simulink model "M10B39_es_V2"  (R2025a)
settings: Solver=ode23tb  StartTime=0.0  StopTime=30  FixedStep=0.001  MaxStep=0.01  RelTol=1e-3  EnableMultiTasking=on
InitFcn:
  | initAll_V2
values from neighbouring files (symbols this model uses):
  acom = 100    [initAll_V1.m]    (also in initAll_V2.m; initAll_V3.m; parameterinit.mat)
  AVm0 = [4.26082678503 4.656135219]    [parameterinit.mat]
  bcom = 50    [initAll_V1.m]    (also in initAll_V2.m; initAll_V3.m; parameterinit.mat)
  busdata = [ ... (first row only)    [PowerFlowData.m]    (also in parameterinit.mat = [1 2 3 4 5 6 7 8 9 10 11 12 ... (585 elements, 39x15)])
  commun = 0*commun    [initAll_V1.m]    (also in initAll_V2.m; initAll_V3.m; parameterinit.mat = [0  0  0; 0  0  0; 0  0  0; 0  0  0])
  Currentin_idx = [8 21 30:39]    [initAll_V2.m]    (also in parameterinit.mat = [8 21 30 31 32 33 34 35 36 37 38 39])
  DataDelay = 0.0*DataDelay    [initAll_V1.m]    (also in initAll_V2.m; initAll_V3.m; parameterinit.mat = [0  0  0; 0  0  0; 0  0  0; 0  0  0])
  ESinit =     [parameterinit.mat]
  fB = 50    [initAll.m]    (also in initAll_V1.m; initAll_V2.m; initAll_V3.m; parameterinit.mat)
  Geninit = Generator_init(opdata,SynMach_in_gidx)    [initAll.m]    (also in initAll_V1.m; initAll_V2.m; initAll_V3.m = Generator_init(opdata_all,SynMach_in_gidx1); parameterinit.mat = )
  lam = 100    [initAll_V1.m]    (also in initAll_V2.m; initAll_V3.m; parameterinit.mat)
  linedata = [1   2 0.00350  0.04110 0.69870 0.0000 ... (first row only)    [PowerFlowData.m]    (also in parameterinit.mat = [1 1 2 2 2 3 3 4 4 5 6 6 ... (276 elements, 46x6)])
  SgridB = 100    [initAll.m]    (also in initAll_V1.m; initAll_V2.m; initAll_V3.m; parameterinit.mat)
  wB = 2*pi*fB    (= 314.159265359)    [initAll.m]    (also in initAll_V1.m; initAll_V2.m; initAll_V3.m; parameterinit.mat)
  Windinit =     [parameterinit.mat]
  YY_load = [3.65450097002 -2.05705688056 0 0 0 0 0 0 0 0 0 0 ... (1521 elements, 39x39)]    [parameterinit.mat]    (also in powerflowcaculate.m = full(YY))
undefined symbols (not defined in the file or in its folder): c1, c2, c3, c4, c5, c6, cp_nom, lambda_nom, P_wind_base, Pelec_base, Pnom
libraries: spsBistableLib x12, simulink_extras x2, simulink x1
(part 2 of 7)

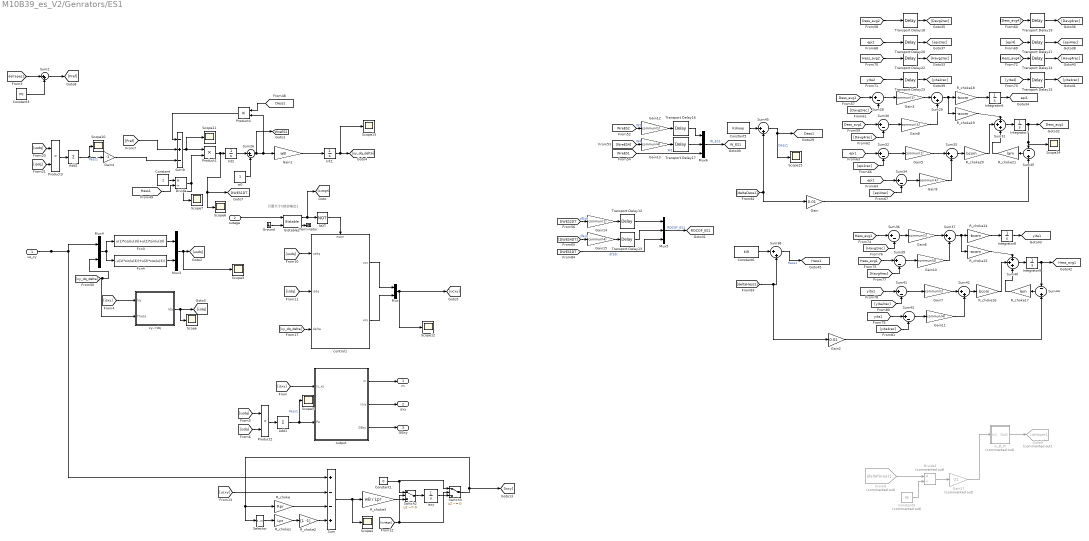
== system M10B39_es_V2/Genrators/ES1 ==
  note: 只要大于0就会输出1
  us_xy : Inport
  outage : Inport  Port=2
  " control1" : Subsystem
  Add1 : Sum  Inputs=+
  Add2 : Sum  Inputs=+
  Bistable2 : spsBistableLib/Bistable  Qpriority=Set  ic=0  Ts=0
  Constant : Constant
  Constant1 : Constant  Value=0
  Constant3 : Constant  Value=P0
  Constant4 : Constant  Commented=on  Value=fB
  Constant5 : Constant  Value=Kdroop
  Constant6 : Constant  Value=KIR
  Divide : Product  Inputs=*/
  Divide2 : Product  Commented=on  Inputs=*/
  Fcn3 : Fcn  Expr=u(1)*cos(u(3))+u(2)*sin(u(3))
  Fcn4 : Fcn  Expr=-u(1)*sin(u(3))+u(2)*cos(u(3))
  From9 : From  Commented=on  GotoTag=deltafarea1  TagVisibility=global
  Gain : Gain  Gain=0.01
  Gain1 : Gain  Gain=wB  SaturateOnIntegerOverflow=on  OutDataTypeStr=Inherit: Same as input  ParamDataTypeStr=Inherit: Same as input
  Gain{8..11,13,15} (6 alike) : Gain  Gain=commun(4)
  Gain{3,5..7,12,14} (6 alike) : Gain  Gain=commun(1)
  Gain17 : Gain  Commented=on  Gain=-21
  Gain2 : Gain  Gain=0.01
  Gain4 : Gain  Gain=-1
  Goto9 : Goto  Commented=on  GotoTag=deltapes1
  Ground : Ground
  Int1 : Integrator  InitialCondition=Dels_hvdc
  Int2 : Integrator  InitialCondition=1
  Integrator{6..9} (4 alike) : Integrator
  Isxy : Integrator  InitialCondition=[Is_xA_0 Is_yA_0]
  Mux : Mux  Inputs=2
  Mux3 : Mux  Inputs=2
  Mux4 : Mux  Inputs=2
  Mux5 : Mux  Inputs=3
  Mux6 : Mux  Inputs=3
  NOT : Logic  Operator=NOT  AllPortsSameDT=off  OutDataTypeStr=boolean
  Product1 : Product
  Product2 : Product  RndMeth=Zero
  Product3 : Product  RndMeth=Zero
  Product4 : Product
  R_choke : Gain  Gain=Rpr  SaturateOnIntegerOverflow=on  OutDataTypeStr=Inherit: Same as input  ParamDataTypeStr=Inherit: Same as input
  R_choke1 : Gain  Gain=Lpr  SaturateOnIntegerOverflow=on  OutDataTypeStr=Inherit: Same as input  ParamDataTypeStr=Inherit: Same as input
  R_choke14 : Gain  Gain=-bcom  SaturateOnIntegerOverflow=on  OutDataTypeStr=Inherit: Same as input  ParamDataTypeStr=Inherit: Same as input
  R_choke15 : Gain  Gain=-acom  SaturateOnIntegerOverflow=on  OutDataTypeStr=Inherit: Same as input  ParamDataTypeStr=Inherit: Same as input
  R_choke16 : Gain  Gain=bcom  SaturateOnIntegerOverflow=on  OutDataTypeStr=Inherit: Same as input  ParamDataTypeStr=Inherit: Same as input
  R_choke17 : Gain  Gain=lam  SaturateOnIntegerOverflow=on  OutDataTypeStr=Inherit: Same as input  ParamDataTypeStr=Inherit: Same as input
  R_choke18 : Gain  Gain=-bcom  SaturateOnIntegerOverflow=on  OutDataTypeStr=Inherit: Same as input  ParamDataTypeStr=Inherit: Same as input
  R_choke19 : Gain  Gain=-acom  SaturateOnIntegerOverflow=on  OutDataTypeStr=Inherit: Same as input  ParamDataTypeStr=Inherit: Same as input
  R_choke2 : Gain  Gain=[1 -1]  SaturateOnIntegerOverflow=on  OutDataTypeStr=Inherit: Same as input  ParamDataTypeStr=Inherit: Same as input
  R_choke20 : Gain  Gain=bcom  SaturateOnIntegerOverflow=on  OutDataTypeStr=Inherit: Same as input  ParamDataTypeStr=Inherit: Same as input
  R_choke21 : Gain  Gain=lam  SaturateOnIntegerOverflow=on  OutDataTypeStr=Inherit: Same as input  ParamDataTypeStr=Inherit: Same as input
  R_choke3 : Gain  Gain=wB / Lpr  SaturateOnIntegerOverflow=on  OutDataTypeStr=Inherit: Same as input  ParamDataTypeStr=Inherit: Same as input
  Scope{,3..7,10..15} (12 alike) : Scope
      Scope settings: ActiveDisplayYMinimum=-0.0194  ActiveDisplayYMaximum=0.04689
      Scope10 settings: ActiveDisplayYMinimum=-0.6053  ActiveDisplayYMaximum=0.06726
      Scope11 settings: ActiveDisplayYMinimum=-0.1125  ActiveDisplayYMaximum=0.0125  DataLoggingVariableName=ScopeData2
      Scope12 settings: ActiveDisplayYMinimum=0.46883  ActiveDisplayYMaximum=1.25548  DataLoggingVariableName=ScopeData3
      Scope13 settings: ActiveDisplayYMinimum=-4.33823  ActiveDisplayYMaximum=0.36599  DataLoggingVariableName=ScopeData4
      Scope14 settings: ActiveDisplayYMinimum=-0.0418  ActiveDisplayYMaximum=0.37621  DataLoggingVariableName=ScopeData2
      Scope15 settings: ActiveDisplayYMinimum=-1  ActiveDisplayYMaximum=1  DataLoggingVariableName=ScopeData3
      Scope3 settings: ActiveDisplayYMinimum=-0.14332  ActiveDisplayYMaximum=1.14443
      Scope4 settings: ActiveDisplayYMinimum=-2.8E-5  ActiveDisplayYMaximum=2.4E-5  DataLoggingVariableName=ScopeData5
      Scope5 settings: ActiveDisplayYMinimum=-0.57271  ActiveDisplayYMaximum=0.19884  DataLoggingVariableName=ScopeData7
      Scope6 settings: ActiveDisplayYMinimum=-0.00021  ActiveDisplayYMaximum=0.0004  DataLoggingVariableName=ScopeData4
      Scope7 settings: ActiveDisplayYMinimum=0.9  ActiveDisplayYMaximum=1.1  DataLoggingVariableName=ScopeData14
  Selector : Selector  InputPortWidth=2  IndexOptions=Index vector (dialog)  Indices=[2 1]  OutputSizes=1
  Sum : Sum  Inputs=+--+  SaturateOnIntegerOverflow=on
  Sum2 : Sum  Inputs=|++
  Sum{26,28,30,32,34,36,39,41,43} (9 alike) : Sum  Inputs=|+-  SaturateOnIntegerOverflow=on
  Sum{29,33,37..38,42,45} (6 alike) : Sum  Inputs=|++  SaturateOnIntegerOverflow=on
  Sum31 : Sum  Inputs=+++  SaturateOnIntegerOverflow=on
  Sum35 : Sum  Inputs=-+  SaturateOnIntegerOverflow=on
  Sum40 : Sum  Inputs=+++  SaturateOnIntegerOverflow=on
  Sum44 : Sum  Inputs=-+  SaturateOnIntegerOverflow=on
  Sum9 : Sum  Inputs=-+-  SaturateOnIntegerOverflow=on
  Switch2 : Switch  Criteria=u2 ~= 0  Threshold=0.5  InputSameDT=off
  Switch3 : Switch  Criteria=u2 ~= 0  Threshold=0.5  InputSameDT=off
  Terminator : Terminator
  Transport Delay{12,16,18,20,22..23} (6 alike) : TransportDelay  DelayTime=DataDelay(2,1)
  Transport Delay{13..15,17,19,21} (6 alike) : TransportDelay  DelayTime=DataDelay(4,2)
  in_D_PI : Subsystem  Commented=on  mask{KP_=0.1, KI_=0.1, Upper_limit=inf, Lower_limit=-inf, Upper_saturation_limit=inf, Lower_saturation_limit=-inf, integrator_init=Md_A_0}
      mask prompts: KP_ "比例系数P"; KI_ "积分系数I"; Upper_limit "限幅上限"; Lower_limit "限幅下限"; Upper_saturation_limit "积分饱和上限"; Lower_saturation_limit "积分饱和下限"; integrator_init "积分初始值"
      mask DialogControl Container4 Prompt: 控制参数
      mask DialogControl Container5 Prompt: 初始值
      mask Display: disp('PI')
  output : Subsystem
  w0 : Constant
  xy->dq : Subsystem
  m : Outport
  isxy : Outport  Port=2
  GBxy : Outport  Port=3
  tag scope: DWES1DT=global, Dess1=global, Dess_avg1=global, Hess1=global, Hess_avg1=global, ROCOF_ES1=global, W_ES1=global, WreES1=global, epi1=global, yita1=global
  wires:
  Selector/1 -> R_choke1/1
  Sum/1 -> Scope4/1, R_choke3/1
  R_choke3/1 -> Switch2/3
  Ground/1 -> Bistable2/2
  R_choke2/1 -> Sum/4
  R_choke/1 -> Sum/3
  [ucxy] -> Sum/2
  output/1(m) -> m/1
  NOT/1 -> " control1"/Enable
  R_choke1/1 -> R_choke2/1
  Bistable2/1 -> NOT/1, [outage]
  Isxy/1 -> Switch3/3
  [isxy] -> xy->dq/1(Ixy)
  [isxy] -> output/1(is_xy)
  output/2(isxy) -> isxy/1
  [xy_dq_delta] -> " control1"/3(delta)
  xy->dq/1(Idq) -> [isdq], Scope/1
  Bistable2/2 -> Terminator/1
  outage/1 -> Bistable2/1
  [outage] -> Switch2/2, Switch3/2
  [isdq] -> " control1"/2(isdq)
  " control1"/1(ucx) -> Mux/1
  Switch2/1 -> Isxy/1
  Switch3/1 -> R_choke/1, Selector/1, [isxy]
  Mux/1 -> Scope12/1, [ucxy]
  [usdq] -> " control1"/1(usdq)
  output/3(GBxy) -> GBxy/1
  Constant1/1 -> Switch2/1, Switch3/1
  " control1"/2(ucy) -> Mux/2
  [usdq] -> Product2/1
  Add1/1 -> Scope5/1, output/2(Pe)  "Pess1"
  Product2/1 -> Add1/1
  [isdq] -> Product2/2
  Product1/1 -> Scope6/1, [DWES1DT], Int2/1
  Sum26/1 -> [WreES1], Product4/2, Gain1/1
  Int2/1 -> Sum26/1
  w0/1 -> Sum26/2
  Sum9/1 -> Product1/1, Scope11/1
  Constant/1 -> Divide/1
  Divide/1 -> Product1/2, Scope7/1
  [Hess1] -> Divide/2
  us_xy/1 -> Mux4/1, Sum/1
  Fcn3/1 -> Mux3/1
  Fcn4/1 -> Mux3/2
  Mux4/1 -> Fcn3/1, Fcn4/1
  [xy_dq_delta] -> Mux4/2, xy->dq/2(Theta)
  Mux3/1 -> Scope3/1, [usdq]
  Gain4/1 -> Sum9/3
  Product4/1 -> Sum9/1
  Int1/1 -> Scope13/1, [xy_dq_delta]
  Add2/1 -> Gain4/1, Scope10/1  "Pess1"
  [usdq] -> Product3/1
  [isdq] -> Product3/2
  Product3/1 -> Add2/1
  Transport Delay19/1 -> [Davg4rec]
  R_choke20/1 -> Sum31/2
  R_choke19/1 -> Sum31/1
  [Dess_avg1] -> Sum28/1
  Transport Delay13/1 -> Mux5/2
  Transport Delay12/1 -> Mux5/1
  [Dess_avg1] -> Sum30/1
  Mux6/1 -> [W_ES1]  "W_ES1"
  [WreES1] -> Mux6/3  "W1"
  Sum38/1 -> [Hess1]  "Hess1"
  Constant5/1 -> Sum45/1
  Sum45/1 -> Scope15/1, [Dess1]  "Dess1"
  Constant6/1 -> Sum38/1
  [epi1] -> Sum34/1
  R_choke21/1 -> Sum31/3
  Integrator6/1 -> [epi1]
  Sum35/1 -> R_choke21/1
  Sum31/1 -> Integrator7/1
  Integrator7/1 -> [Dess_avg1], Scope14/1, Sum35/1
  Transport Delay21/1 -> [epi4rec]
  [epi2] -> Transport Delay20/1
  [epi4rec] -> Sum34/2
  [DWES1DT] -> Mux5/3  "df1dt"
  [Davg4rec] -> Sum30/2
  [yita2rec] -> Sum41/2
  [yita1] -> Sum41/1
  Sum40/1 -> Integrator9/1
  [deltaDess1] -> Sum45/2, Gain/1
  R_choke18/1 -> Integrator6/1
  [Havg4rec] -> Sum39/2
  [epi1] -> Sum32/1
  [Havg2rec] -> Sum36/2
  Sum42/1 -> R_choke16/1
  [Dess_avg2] -> Transport Delay18/1
  Transport Delay20/1 -> [epi2rec]
  Transport Delay14/1 -> [Havg4rec]
  [Hess_avg1] -> Sum39/1
  Mux5/1 -> [ROCOF_ES1]  "ROCOF_ES1"
  Integrator9/1 -> [Hess_avg1], Sum44/1
  Sum29/1 -> R_choke19/1, R_choke18/1
  [Davg2rec] -> Sum28/2
  [yita2] -> Transport Delay23/1
  Sum37/1 -> R_choke15/1, R_choke14/1
  R_choke14/1 -> Integrator8/1
  Integrator8/1 -> [yita1]
  Transport Delay18/1 -> [Davg2rec]
  R_choke17/1 -> Sum40/3
  Transport Delay17/1 -> Mux6/2
  R_choke15/1 -> Sum40/1
  R_choke16/1 -> Sum40/2
  [Hess_avg1] -> Sum36/1
  [deltaHess1] -> Sum38/2, Gain2/1
  Sum44/1 -> R_choke17/1
  Sum33/1 -> R_choke20/1
  Transport Delay23/1 -> [yita2rec]
  Transport Delay16/1 -> Mux6/1
  [epi2rec] -> Sum32/2
  Transport Delay22/1 -> [Havg2rec]
  Transport Delay15/1 -> [yita4rec]
  [Hess_avg2] -> Transport Delay22/1
  [Dess1] -> Product4/1
  Gain1/1 -> Int1/1
  [yita4rec] -> Sum43/2
  [yita1] -> Sum43/1
  Gain/1 -> Sum35/2
  Gain2/1 -> Sum44/2
  [Dess_avg4] -> Transport Delay19/1
  [epi4] -> Transport Delay21/1
  [Hess_avg4] -> Transport Delay14/1
  [yita4] -> Transport Delay15/1
  [WreES2] -> Gain12/1  "W2"
  Gain12/1 -> Transport Delay16/1
  [WreES4] -> Gain13/1  "W4"
  Gain13/1 -> Transport Delay17/1
  [DWES2DT] -> Gain14/1  "df2dt"
  Gain14/1 -> Transport Delay12/1
  [DWES4DT] -> Gain15/1  "df4dt"
  Gain15/1 -> Transport Delay13/1
  Gain3/1 -> Sum29/1
  Sum28/1 -> Gain3/1
  Gain5/1 -> Sum33/1
  Sum32/1 -> Gain5/1
  Sum36/1 -> Gain6/1
  Gain6/1 -> Sum37/1
  Gain7/1 -> Sum42/1
  Sum41/1 -> Gain7/1
  Sum30/1 -> Gain8/1
  Gain8/1 -> Sum29/2
  Sum34/1 -> Gain9/1
  Gain9/1 -> Sum33/2
  Sum39/1 -> Gain10/1
  Gain10/1 -> Sum37/2
  Sum43/1 -> Gain11/1
  Gain11/1 -> Sum42/2
  [deltapes1] -> Sum2/1
  Sum2/1 -> [Pref]
  Constant3/1 -> Sum2/2
  [Pref] -> Sum9/2
  Divide2/1 -> Gain17/1
  Constant4/1 -> Divide2/2
  From9/1 -> Divide2/1
  in_D_PI/1(Out1) -> Goto9/1
  Gain17/1 -> in_D_PI/1(In1)

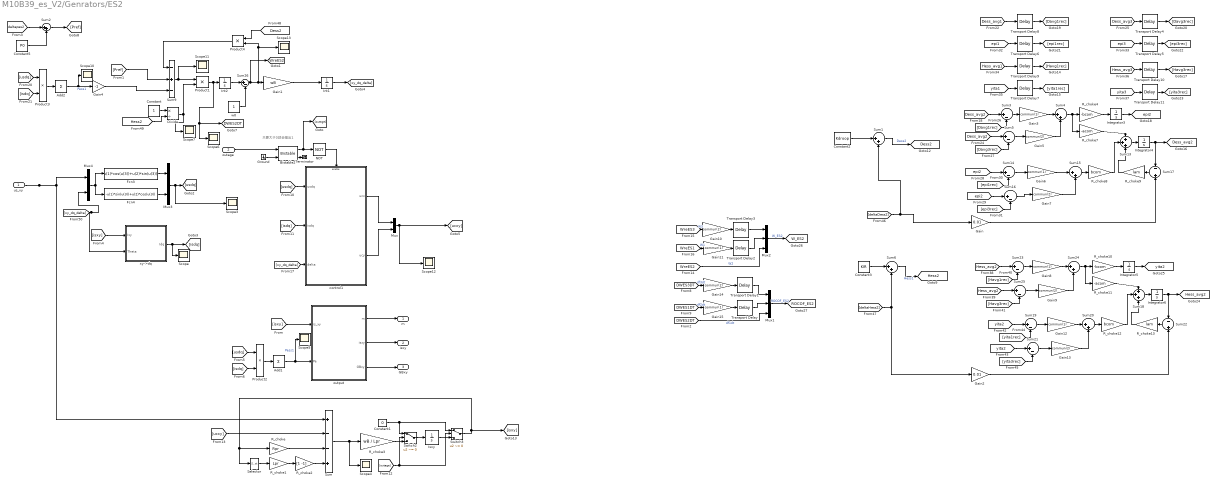
== system M10B39_es_V2/Genrators/ES2 ==
  note: 只要大于0就会输出1
  us_xy : Inport
  outage : Inport  Port=2
  " control1" : Subsystem
  Add1 : Sum  Inputs=+
  Add2 : Sum  Inputs=+
  Bistable2 : spsBistableLib/Bistable  Qpriority=Set  ic=0  Ts=0
  Constant : Constant
  Constant1 : Constant  Value=0
  Constant2 : Constant  Value=Kdroop
  Constant3 : Constant  Value=KIR
  Constant5 : Constant  Value=P0
  Divide : Product  Inputs=*/
  Fcn3 : Fcn  Expr=u(1)*cos(u(3))+u(2)*sin(u(3))
  Fcn4 : Fcn  Expr=-u(1)*sin(u(3))+u(2)*cos(u(3))
  Gain : Gain  Gain=0.01
  Gain1 : Gain  Gain=wB  SaturateOnIntegerOverflow=on  OutDataTypeStr=Inherit: Same as input  ParamDataTypeStr=Inherit: Same as input
  Gain{5,7,9..10,13..14} (6 alike) : Gain  Gain=commun(2)
  Gain{3,6,8,11..12,15} (6 alike) : Gain  Gain=commun(1)
  Gain2 : Gain  Gain=0.01
  Gain4 : Gain  Gain=-1
  Ground : Ground
  Int1 : Integrator  InitialCondition=Dels_hvdc
  Int2 : Integrator  InitialCondition=1
  Integrator{3..6} (4 alike) : Integrator
  Isxy : Integrator  InitialCondition=[Is_xA_0 Is_yA_0]
  Mux : Mux  Inputs=2
  Mux1 : Mux  Inputs=3
  Mux2 : Mux  Inputs=3
  Mux3 : Mux  Inputs=2
  Mux4 : Mux  Inputs=2
  NOT : Logic  Operator=NOT  AllPortsSameDT=off  OutDataTypeStr=boolean
  Product1 : Product
  Product2 : Product  RndMeth=Zero
  Product3 : Product  RndMeth=Zero
  Product4 : Product
  R_choke : Gain  Gain=Rpr  SaturateOnIntegerOverflow=on  OutDataTypeStr=Inherit: Same as input  ParamDataTypeStr=Inherit: Same as input
  R_choke1 : Gain  Gain=Lpr  SaturateOnIntegerOverflow=on  OutDataTypeStr=Inherit: Same as input  ParamDataTypeStr=Inherit: Same as input
  R_choke10 : Gain  Gain=-bcom  SaturateOnIntegerOverflow=on  OutDataTypeStr=Inherit: Same as input  ParamDataTypeStr=Inherit: Same as input
  R_choke11 : Gain  Gain=-acom  SaturateOnIntegerOverflow=on  OutDataTypeStr=Inherit: Same as input  ParamDataTypeStr=Inherit: Same as input
  R_choke12 : Gain  Gain=bcom  SaturateOnIntegerOverflow=on  OutDataTypeStr=Inherit: Same as input  ParamDataTypeStr=Inherit: Same as input
  R_choke13 : Gain  Gain=lam  SaturateOnIntegerOverflow=on  OutDataTypeStr=Inherit: Same as input  ParamDataTypeStr=Inherit: Same as input
  R_choke2 : Gain  Gain=[1 -1]  SaturateOnIntegerOverflow=on  OutDataTypeStr=Inherit: Same as input  ParamDataTypeStr=Inherit: Same as input
  R_choke3 : Gain  Gain=wB / Lpr  SaturateOnIntegerOverflow=on  OutDataTypeStr=Inherit: Same as input  ParamDataTypeStr=Inherit: Same as input
  R_choke4 : Gain  Gain=-bcom  SaturateOnIntegerOverflow=on  OutDataTypeStr=Inherit: Same as input  ParamDataTypeStr=Inherit: Same as input
  R_choke7 : Gain  Gain=-acom  SaturateOnIntegerOverflow=on  OutDataTypeStr=Inherit: Same as input  ParamDataTypeStr=Inherit: Same as input
  R_choke8 : Gain  Gain=bcom  SaturateOnIntegerOverflow=on  OutDataTypeStr=Inherit: Same as input  ParamDataTypeStr=Inherit: Same as input
  R_choke9 : Gain  Gain=lam  SaturateOnIntegerOverflow=on  OutDataTypeStr=Inherit: Same as input  ParamDataTypeStr=Inherit: Same as input
  Scope{,3..7,10..13} (10 alike) : Scope
      Scope settings: ActiveDisplayYMinimum=-0.0194  ActiveDisplayYMaximum=0.04689
      Scope10 settings: ActiveDisplayYMinimum=-0.00511  ActiveDisplayYMaximum=0.046
      Scope11 settings: ActiveDisplayYMinimum=-0.1125  ActiveDisplayYMaximum=0.0125  DataLoggingVariableName=ScopeData2
      Scope12 settings: ActiveDisplayYMinimum=0.46883  ActiveDisplayYMaximum=1.25548  DataLoggingVariableName=ScopeData3
      Scope13 settings: ActiveDisplayYMinimum=-0.0063  ActiveDisplayYMaximum=0.05669  DataLoggingVariableName=ScopeData4
      Scope3 settings: ActiveDisplayYMinimum=-0.12696  ActiveDisplayYMaximum=1.14248
      Scope4 settings: ActiveDisplayYMinimum=-2.8E-5  ActiveDisplayYMaximum=2.4E-5  DataLoggingVariableName=ScopeData5
      Scope5 settings: ActiveDisplayYMinimum=-0.00823  ActiveDisplayYMaximum=0.07404  DataLoggingVariableName=ScopeData7
      Scope6 settings: ActiveDisplayYMinimum=-0.00105  ActiveDisplayYMaximum=0.00091  DataLoggingVariableName=ScopeData4
      Scope7 settings: ActiveDisplayYMinimum=0.9  ActiveDisplayYMaximum=1.1  DataLoggingVariableName=ScopeData14
  Selector : Selector  InputPortWidth=2  IndexOptions=Index vector (dialog)  Indices=[2 1]  OutputSizes=1
  Sum : Sum  Inputs=+--+  SaturateOnIntegerOverflow=on
  Sum{1,4,6,15,20,24} (6 alike) : Sum  Inputs=|++  SaturateOnIntegerOverflow=on
  Sum13 : Sum  Inputs=+++  SaturateOnIntegerOverflow=on
  Sum{3,5,14,16,19,21,23,25..26} (9 alike) : Sum  Inputs=|+-  SaturateOnIntegerOverflow=on
  Sum17 : Sum  Inputs=-+  SaturateOnIntegerOverflow=on
  Sum18 : Sum  Inputs=+++  SaturateOnIntegerOverflow=on
  Sum2 : Sum  Inputs=|++
  Sum22 : Sum  Inputs=-+  SaturateOnIntegerOverflow=on
  Sum9 : Sum  Inputs=-+-  SaturateOnIntegerOverflow=on
  Switch2 : Switch  Criteria=u2 ~= 0  Threshold=0.5  InputSameDT=off
  Switch3 : Switch  Criteria=u2 ~= 0  Threshold=0.5  InputSameDT=off
  Terminator : Terminator
  Transport Delay{,2,6..9} (6 alike) : TransportDelay  DelayTime=DataDelay(1,2)
  Transport Delay{1,3..5,10..11} (6 alike) : TransportDelay  DelayTime=DataDelay(3,1)
  output : Subsystem
  w0 : Constant
  xy->dq : Subsystem
  m : Outport
  isxy : Outport  Port=2
  GBxy : Outport  Port=3
  tag scope: DWES2DT=global, Dess2=global, Dess_avg2=global, Hess2=global, Hess_avg2=global, ROCOF_ES2=global, W_ES2=global, WreES2=global, epi2=global, yita2=global
  wires:
  Selector/1 -> R_choke1/1
  Sum/1 -> Scope4/1, R_choke3/1
  R_choke3/1 -> Switch2/3
  Ground/1 -> Bistable2/2
  R_choke2/1 -> Sum/4
  R_choke/1 -> Sum/3
  [ucxy] -> Sum/2
  output/1(m) -> m/1
  NOT/1 -> " control1"/Enable
  R_choke1/1 -> R_choke2/1
  Bistable2/1 -> NOT/1, [outage]
  Isxy/1 -> Switch3/3
  [isxy] -> xy->dq/1(Ixy)
  [isxy] -> output/1(is_xy)
  output/2(isxy) -> isxy/1
  [xy_dq_delta] -> " control1"/3(delta)
  xy->dq/1(Idq) -> [isdq], Scope/1
  Bistable2/2 -> Terminator/1
  outage/1 -> Bistable2/1
  [outage] -> Switch2/2, Switch3/2
  [isdq] -> " control1"/2(isdq)
  " control1"/1(ucx) -> Mux/1
  Switch2/1 -> Isxy/1
  Switch3/1 -> R_choke/1, Selector/1, [isxy]
  Mux/1 -> Scope12/1, [ucxy]
  [usdq] -> " control1"/1(usdq)
  output/3(GBxy) -> GBxy/1
  Constant1/1 -> Switch2/1, Switch3/1
  " control1"/2(ucy) -> Mux/2
  [usdq] -> Product2/1
  Add1/1 -> Scope5/1, output/2(Pe)  "Pess1"
  Product2/1 -> Add1/1
  [isdq] -> Product2/2
  Product1/1 -> Scope6/1, [DWES2DT], Int2/1
  Sum26/1 -> [WreES2], Scope13/1, Product4/2, Gain1/1
  Int2/1 -> Sum26/1
  w0/1 -> Sum26/2
  Sum9/1 -> Product1/1, Scope11/1
  Constant/1 -> Divide/1
  Divide/1 -> Product1/2, Scope7/1
  [Hess2] -> Divide/2
  us_xy/1 -> Mux4/1, Sum/1
  Fcn3/1 -> Mux3/1
  Fcn4/1 -> Mux3/2
  Mux4/1 -> Fcn3/1, Fcn4/1
  [xy_dq_delta] -> Mux4/2, xy->dq/2(Theta)
  Mux3/1 -> Scope3/1, [usdq]
  Gain4/1 -> Sum9/3
  Product4/1 -> Sum9/1
  Int1/1 -> [xy_dq_delta]
  Add2/1 -> Gain4/1, Scope10/1  "Pess1"
  [usdq] -> Product3/1
  [isdq] -> Product3/2
  Product3/1 -> Add2/1
  [Dess2] -> Product4/1
  Gain1/1 -> Int1/1
  [Davg3rec] -> Sum5/2
  R_choke7/1 -> Sum13/1
  [yita1rec] -> Sum19/2
  Transport Delay/1 -> Mux1/2
  R_choke8/1 -> Sum13/2
  [Dess_avg2] -> Sum5/1
  [Dess_avg2] -> Sum3/1
  Transport Delay9/1 -> [Havg1rec]
  [Davg1rec] -> Sum3/2
  Transport Delay6/1 -> [epi1rec]
  [WreES2] -> Mux2/3  "W2"
  Integrator3/1 -> [epi2]
  [epi1rec] -> Sum14/2
  Transport Delay5/1 -> [epi3rec]
  Mux1/1 -> [ROCOF_ES2]  "ROCOF_ES2"
  Sum20/1 -> R_choke12/1
  Transport Delay4/1 -> [Davg3rec]
  [yita2] -> Sum21/1
  Transport Delay7/1 -> [yita1rec]
  Transport Delay3/1 -> Mux2/1
  Sum17/1 -> R_choke9/1
  [deltaDess2] -> Gain/1, Sum1/2
  [Hess_avg2] -> Sum25/1
  Sum13/1 -> Integrator4/1
  R_choke10/1 -> Integrator5/1
  Sum15/1 -> R_choke8/1
  R_choke9/1 -> Sum13/3
  Constant3/1 -> Sum6/1
  Integrator4/1 -> [Dess_avg2], Sum17/1
  [epi2] -> Sum16/1
  [deltaHess2] -> Sum6/2, Gain2/1
  Transport Delay10/1 -> [Havg3rec]
  [epi3rec] -> Sum16/2
  Sum24/1 -> R_choke11/1, R_choke10/1
  [DWES2DT] -> Mux1/3  "df1dt"
  Sum6/1 -> [Hess2]  "Hess1"
  [yita2] -> Sum19/1
  Transport Delay1/1 -> Mux1/1
  [epi2] -> Sum14/1
  R_choke12/1 -> Sum18/2
  [Hess_avg2] -> Sum23/1
  R_choke11/1 -> Sum18/1
  Transport Delay2/1 -> Mux2/2
  R_choke4/1 -> Integrator3/1
  Mux2/1 -> [W_ES2]  "W_ES2"
  Sum4/1 -> R_choke7/1, R_choke4/1
  [yita3rec] -> Sum21/2
  [Havg1rec] -> Sum23/2
  [Havg3rec] -> Sum25/2
  Transport Delay11/1 -> [yita3rec]
  Sum22/1 -> R_choke13/1
  Integrator6/1 -> [Hess_avg2], Sum22/1
  Sum18/1 -> Integrator6/1
  Integrator5/1 -> [yita2]
  R_choke13/1 -> Sum18/3
  Transport Delay8/1 -> [Davg1rec]
  Sum1/1 -> [Dess2]  "Dess2"
  Constant2/1 -> Sum1/1
  Gain/1 -> Sum17/2
  Gain2/1 -> Sum22/2
  [Dess_avg1] -> Transport Delay8/1
  [epi1] -> Transport Delay6/1
  [Hess_avg1] -> Transport Delay9/1
  [yita1] -> Transport Delay7/1
  [Dess_avg3] -> Transport Delay4/1
  [epi3] -> Transport Delay5/1
  [Hess_avg3] -> Transport Delay10/1
  [yita3] -> Transport Delay11/1
  [WreES3] -> Gain10/1  "W3"
  Gain10/1 -> Transport Delay3/1
  [WreES1] -> Gain11/1  "W1"
  Gain11/1 -> Transport Delay2/1
  [DWES3DT] -> Gain14/1  "df3dt"
  Gain14/1 -> Transport Delay1/1
  [DWES1DT] -> Gain15/1  "df2dt"
  Gain15/1 -> Transport Delay/1
  Gain3/1 -> Sum4/1
  Sum3/1 -> Gain3/1
  Sum5/1 -> Gain5/1
  Gain5/1 -> Sum4/2
  Gain6/1 -> Sum15/1
  Sum14/1 -> Gain6/1
  Sum16/1 -> Gain7/1
  Gain7/1 -> Sum15/2
  Sum23/1 -> Gain8/1
  Gain8/1 -> Sum24/1
  Sum25/1 -> Gain9/1
  Gain9/1 -> Sum24/2
  Gain12/1 -> Sum20/1
  Sum19/1 -> Gain12/1
  Sum21/1 -> Gain13/1
  Gain13/1 -> Sum20/2
  Constant5/1 -> Sum2/2
  Sum2/1 -> [Pref]
  [deltapes2] -> Sum2/1
  [Pref] -> Sum9/2

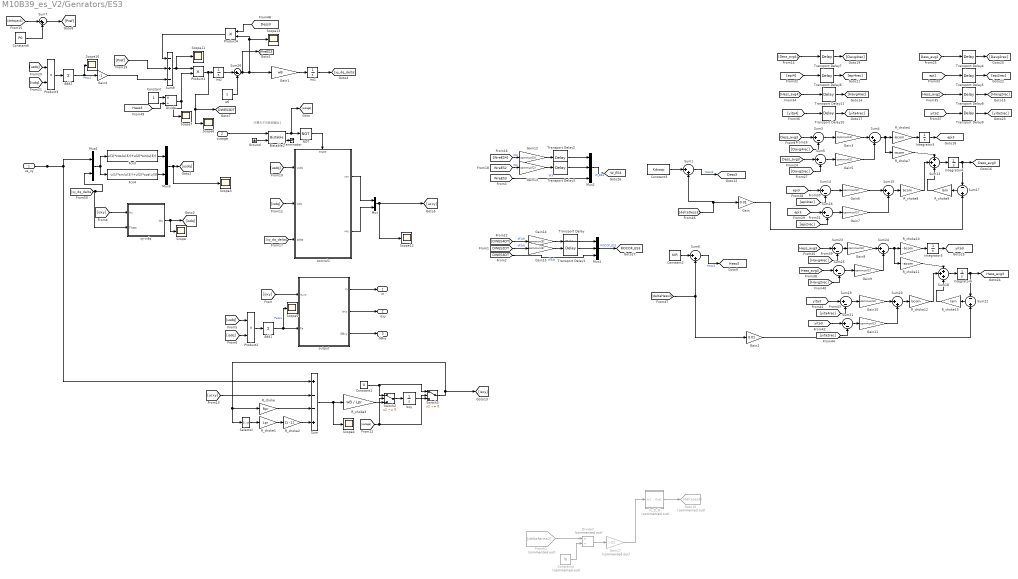
== system M10B39_es_V2/Genrators/ES3 ==
  note: 只要大于0就会输出1
  us_xy : Inport
  outage : Inport  Port=2
  " control1" : Subsystem
  Add1 : Sum  Inputs=+
  Add2 : Sum  Inputs=+
  Bistable2 : spsBistableLib/Bistable  Qpriority=Set  ic=0  Ts=0
  Constant : Constant
  Constant1 : Constant  Value=0
  Constant2 : Constant  Value=KIR
  Constant3 : Constant  Value=Kdroop
  Constant4 : Constant  Commented=on  Value=fB
  Constant6 : Constant  Value=P0
  Divide : Product  Inputs=*/
  Divide2 : Product  Commented=on  Inputs=*/
  Fcn3 : Fcn  Expr=u(1)*cos(u(3))+u(2)*sin(u(3))
  Fcn4 : Fcn  Expr=-u(1)*sin(u(3))+u(2)*cos(u(3))
  From51 : From  Commented=on  GotoTag=deltafarea2  TagVisibility=global
  Gain : Gain  Gain=0.01
  Gain1 : Gain  Gain=wB  SaturateOnIntegerOverflow=on  OutDataTypeStr=Inherit: Same as input  ParamDataTypeStr=Inherit: Same as input
  Gain{3,6,8,10,12,14} (6 alike) : Gain  Gain=commun(3)
  Gain{5,7,9,11,13,15} (6 alike) : Gain  Gain=commun(2)
  Gain17 : Gain  Commented=on  Gain=-21
  Gain2 : Gain  Gain=0.01
  Gain4 : Gain  Gain=-1
  Goto10 : Goto  Commented=on  GotoTag=deltapes3
  Ground : Ground
  Int1 : Integrator  InitialCondition=Dels_hvdc
  Int2 : Integrator  InitialCondition=1
  Integrator{3..6} (4 alike) : Integrator
  Isxy : Integrator  InitialCondition=[Is_xA_0 Is_yA_0]
  Mux : Mux  Inputs=2
  Mux1 : Mux  Inputs=3
  Mux2 : Mux  Inputs=3
  Mux3 : Mux  Inputs=2
  Mux4 : Mux  Inputs=2
  NOT : Logic  Operator=NOT  AllPortsSameDT=off  OutDataTypeStr=boolean
  Product1 : Product
  Product2 : Product  RndMeth=Zero
  Product3 : Product  RndMeth=Zero
  Product4 : Product
  R_choke : Gain  Gain=Rpr  SaturateOnIntegerOverflow=on  OutDataTypeStr=Inherit: Same as input  ParamDataTypeStr=Inherit: Same as input
  R_choke1 : Gain  Gain=Lpr  SaturateOnIntegerOverflow=on  OutDataTypeStr=Inherit: Same as input  ParamDataTypeStr=Inherit: Same as input
  R_choke10 : Gain  Gain=-bcom  SaturateOnIntegerOverflow=on  OutDataTypeStr=Inherit: Same as input  ParamDataTypeStr=Inherit: Same as input
  R_choke11 : Gain  Gain=-acom  SaturateOnIntegerOverflow=on  OutDataTypeStr=Inherit: Same as input  ParamDataTypeStr=Inherit: Same as input
  R_choke12 : Gain  Gain=bcom  SaturateOnIntegerOverflow=on  OutDataTypeStr=Inherit: Same as input  ParamDataTypeStr=Inherit: Same as input
  R_choke13 : Gain  Gain=lam  SaturateOnIntegerOverflow=on  OutDataTypeStr=Inherit: Same as input  ParamDataTypeStr=Inherit: Same as input
  R_choke2 : Gain  Gain=[1 -1]  SaturateOnIntegerOverflow=on  OutDataTypeStr=Inherit: Same as input  ParamDataTypeStr=Inherit: Same as input
  R_choke3 : Gain  Gain=wB / Lpr  SaturateOnIntegerOverflow=on  OutDataTypeStr=Inherit: Same as input  ParamDataTypeStr=Inherit: Same as input
  R_choke4 : Gain  Gain=-bcom  SaturateOnIntegerOverflow=on  OutDataTypeStr=Inherit: Same as input  ParamDataTypeStr=Inherit: Same as input
  R_choke7 : Gain  Gain=-acom  SaturateOnIntegerOverflow=on  OutDataTypeStr=Inherit: Same as input  ParamDataTypeStr=Inherit: Same as input
  R_choke8 : Gain  Gain=bcom  SaturateOnIntegerOverflow=on  OutDataTypeStr=Inherit: Same as input  ParamDataTypeStr=Inherit: Same as input
  R_choke9 : Gain  Gain=lam  SaturateOnIntegerOverflow=on  OutDataTypeStr=Inherit: Same as input  ParamDataTypeStr=Inherit: Same as input
  Scope{,3..7,10..13} (10 alike) : Scope
      Scope settings: ActiveDisplayYMinimum=-0.0194  ActiveDisplayYMaximum=0.04689
      Scope10 settings: ActiveDisplayYMinimum=-0.00511  ActiveDisplayYMaximum=0.046
      Scope11 settings: ActiveDisplayYMinimum=-0.1125  ActiveDisplayYMaximum=0.0125  DataLoggingVariableName=ScopeData2
      Scope12 settings: ActiveDisplayYMinimum=0.46883  ActiveDisplayYMaximum=1.25548  DataLoggingVariableName=ScopeData3
      Scope13 settings: ActiveDisplayYMinimum=-0.00656  ActiveDisplayYMaximum=0.05904  DataLoggingVariableName=ScopeData4
      Scope3 settings: ActiveDisplayYMinimum=-0.12696  ActiveDisplayYMaximum=1.14248
      Scope4 settings: ActiveDisplayYMinimum=-2.8E-5  ActiveDisplayYMaximum=2.4E-5  DataLoggingVariableName=ScopeData5
      Scope5 settings: ActiveDisplayYMinimum=-0.00823  ActiveDisplayYMaximum=0.07404  DataLoggingVariableName=ScopeData7
      Scope6 settings: ActiveDisplayYMinimum=-4.9E-5  ActiveDisplayYMaximum=-0  DataLoggingVariableName=ScopeData4
      Scope7 settings: ActiveDisplayYMinimum=0.9  ActiveDisplayYMaximum=1.1  DataLoggingVariableName=ScopeData14
  Selector : Selector  InputPortWidth=2  IndexOptions=Index vector (dialog)  Indices=[2 1]  OutputSizes=1
  Sum : Sum  Inputs=+--+  SaturateOnIntegerOverflow=on
  Sum{1,4,6,15,20,24} (6 alike) : Sum  Inputs=|++  SaturateOnIntegerOverflow=on
  Sum13 : Sum  Inputs=+++  SaturateOnIntegerOverflow=on
  Sum{3,5,14,16,19,21,23,25..26} (9 alike) : Sum  Inputs=|+-  SaturateOnIntegerOverflow=on
  Sum17 : Sum  Inputs=-+  SaturateOnIntegerOverflow=on
  Sum18 : Sum  Inputs=+++  SaturateOnIntegerOverflow=on
  Sum22 : Sum  Inputs=-+  SaturateOnIntegerOverflow=on
  Sum7 : Sum  Inputs=|++
  Sum9 : Sum  Inputs=-+-  SaturateOnIntegerOverflow=on
  Switch2 : Switch  Criteria=u2 ~= 0  Threshold=0.5  InputSameDT=off
  Switch3 : Switch  Criteria=u2 ~= 0  Threshold=0.5  InputSameDT=off
  Terminator : Terminator
  Transport Delay{,2,6..7,10..11} (6 alike) : TransportDelay  DelayTime=DataDelay(4,1)
  Transport Delay{1,3..5,8..9} (6 alike) : TransportDelay  DelayTime=DataDelay(2,2)
  in_D_PI : Subsystem  Commented=on  mask{KP_=0.1, KI_=0.1, Upper_limit=inf, Lower_limit=-inf, Upper_saturation_limit=inf, Lower_saturation_limit=-inf, integrator_init=Md_A_0}
      mask prompts: KP_ "比例系数P"; KI_ "积分系数I"; Upper_limit "限幅上限"; Lower_limit "限幅下限"; Upper_saturation_limit "积分饱和上限"; Lower_saturation_limit "积分饱和下限"; integrator_init "积分初始值"
      mask DialogControl Container4 Prompt: 控制参数
      mask DialogControl Container5 Prompt: 初始值
      mask Display: disp('PI')
  output : Subsystem
  w0 : Constant
  xy->dq : Subsystem
  m : Outport
  isxy : Outport  Port=2
  GBxy : Outport  Port=3
  tag scope: DWES3DT=global, Dess3=global, Dess_avg3=global, Hess3=global, Hess_avg3=global, ROCOF_ES3=global, W_ES3=global, WreES3=global, epi3=global, yita3=global
  wires:
  Selector/1 -> R_choke1/1
  Sum/1 -> Scope4/1, R_choke3/1
  R_choke3/1 -> Switch2/3
  Ground/1 -> Bistable2/2
  R_choke2/1 -> Sum/4
  R_choke/1 -> Sum/3
  [ucxy] -> Sum/2
  output/1(m) -> m/1
  NOT/1 -> " control1"/Enable
  R_choke1/1 -> R_choke2/1
  Bistable2/1 -> NOT/1, [outage]
  Isxy/1 -> Switch3/3
  [isxy] -> xy->dq/1(Ixy)
  [isxy] -> output/1(is_xy)
  output/2(isxy) -> isxy/1
  [xy_dq_delta] -> " control1"/3(delta)
  xy->dq/1(Idq) -> [isdq], Scope/1
  Bistable2/2 -> Terminator/1
  outage/1 -> Bistable2/1
  [outage] -> Switch2/2, Switch3/2
  [isdq] -> " control1"/2(isdq)
  " control1"/1(ucx) -> Mux/1
  Switch2/1 -> Isxy/1
  Switch3/1 -> R_choke/1, Selector/1, [isxy]
  Mux/1 -> Scope12/1, [ucxy]
  [usdq] -> " control1"/1(usdq)
  output/3(GBxy) -> GBxy/1
  Constant1/1 -> Switch2/1, Switch3/1
  " control1"/2(ucy) -> Mux/2
  [usdq] -> Product2/1
  Add1/1 -> Scope5/1, output/2(Pe)  "Pess1"
  Product2/1 -> Add1/1
  [isdq] -> Product2/2
  Product1/1 -> Scope6/1, [DWES3DT], Int2/1
  Int2/1 -> Sum26/1
  w0/1 -> Sum26/2
  Sum9/1 -> Product1/1, Scope11/1
  Constant/1 -> Divide/1
  Divide/1 -> Product1/2, Scope7/1
  [Hess3] -> Divide/2
  us_xy/1 -> Mux4/1, Sum/1
  Fcn3/1 -> Mux3/1
  Fcn4/1 -> Mux3/2
  Mux4/1 -> Fcn3/1, Fcn4/1
  [xy_dq_delta] -> Mux4/2, xy->dq/2(Theta)
  Mux3/1 -> Scope3/1, [usdq]
  Gain4/1 -> Sum9/3
  Product4/1 -> Sum9/1
  Int1/1 -> [xy_dq_delta]
  Add2/1 -> Gain4/1, Scope10/1  "Pess1"
  [usdq] -> Product3/1
  [isdq] -> Product3/2
  Product3/1 -> Add2/1
  [Dess3] -> Product4/1
  Gain1/1 -> Int1/1
  R_choke8/1 -> Sum13/2
  Transport Delay9/1 -> [yita2rec]
  Sum6/1 -> [Hess3]  "Hess3"
  [yita3] -> Sum21/1
  R_choke4/1 -> Integrator3/1
  [WreES3] -> Mux2/3  "W3"
  Transport Delay/1 -> Mux1/1
  [Havg4rec] -> Sum23/2
  [Dess_avg3] -> Sum3/1
  [Havg2rec] -> Sum25/2
  [Dess_avg3] -> Sum5/1
  [Davg2rec] -> Sum5/2
  [DWES3DT] -> Mux1/3  "df3dt"
  Transport Delay4/1 -> [Davg2rec]
  Mux2/1 -> [W_ES3]  "W_ES3"
  [Hess_avg3] -> Sum23/1
  Transport Delay1/1 -> Mux1/2
  Constant2/1 -> Sum6/1
  Sum1/1 -> [Dess3]  "Dess3"
  Constant3/1 -> Sum1/1
  [epi3] -> Sum14/1
  Sum20/1 -> R_choke12/1
  [Davg4rec] -> Sum3/2
  [epi4rec] -> Sum14/2
  [epi3] -> Sum16/1
  R_choke13/1 -> Sum18/3
  Sum24/1 -> R_choke11/1, R_choke10/1
  R_choke7/1 -> Sum13/1
  R_choke9/1 -> Sum13/3
  [yita2rec] -> Sum21/2
  Sum4/1 -> R_choke7/1, R_choke4/1
  R_choke11/1 -> Sum18/1
  Transport Delay5/1 -> [epi2rec]
  Transport Delay2/1 -> Mux2/1
  Integrator5/1 -> [yita3]
  Transport Delay3/1 -> Mux2/2
  Transport Delay10/1 -> [yita4rec]
  [Hess_avg3] -> Sum25/1
  Integrator6/1 -> [Hess_avg3], Sum22/1
  Transport Delay7/1 -> [Davg4rec]
  R_choke10/1 -> Integrator5/1
  Integrator3/1 -> [epi3]
  Transport Delay6/1 -> [epi4rec]
  Transport Delay11/1 -> [Havg4rec]
  Transport Delay8/1 -> [Havg2rec]
  Sum17/1 -> R_choke9/1
  [epi2rec] -> Sum16/2
  Sum22/1 -> R_choke13/1
  Sum15/1 -> R_choke8/1
  [yita4rec] -> Sum19/2
  R_choke12/1 -> Sum18/2
  Sum18/1 -> Integrator6/1
  [deltaDess3] -> Sum1/2, Gain/1
  Mux1/1 -> [ROCOF_ES3]  "ROCOF_ES3"
  Integrator4/1 -> [Dess_avg3], Sum17/1
  Sum13/1 -> Integrator4/1
  [yita3] -> Sum19/1
  Sum26/1 -> [WreES3], Gain1/1, Scope13/1, Product4/2
  Gain/1 -> Sum17/2
  Gain2/1 -> Sum22/2
  [Dess_avg4] -> Transport Delay7/1
  [epi4] -> Transport Delay6/1
  [Hess_avg4] -> Transport Delay11/1
  [yita4] -> Transport Delay10/1
  [yita2] -> Transport Delay9/1
  [Hess_avg2] -> Transport Delay8/1
  [epi2] -> Transport Delay5/1
  [Dess_avg2] -> Transport Delay4/1
  [WreES4] -> Gain12/1  "W4"
  Gain12/1 -> Transport Delay2/1
  [WreES2] -> Gain13/1  "W2"
  Gain13/1 -> Transport Delay3/1
  Gain14/1 -> Transport Delay/1
  [DWES4DT] -> Gain14/1  "df1dt"
  Gain15/1 -> Transport Delay1/1
  [DWES2DT] -> Gain15/1  "df2dt"
  [deltaHess3] -> Gain2/1, Sum6/2
  Gain3/1 -> Sum4/1
  Sum3/1 -> Gain3/1
  Sum5/1 -> Gain5/1
  Gain5/1 -> Sum4/2
  Sum14/1 -> Gain6/1
  Gain6/1 -> Sum15/1
  Sum16/1 -> Gain7/1
  Gain7/1 -> Sum15/2
  Sum23/1 -> Gain8/1
  Gain8/1 -> Sum24/1
  Gain9/1 -> Sum24/2
  Sum25/1 -> Gain9/1
  Sum19/1 -> Gain10/1
  Gain10/1 -> Sum20/1
  Gain11/1 -> Sum20/2
  Sum21/1 -> Gain11/1
  [deltapes3] -> Sum7/1
  Constant6/1 -> Sum7/2
  Sum7/1 -> [Pref]
  [Pref] -> Sum9/2
  From51/1 -> Divide2/1
  Constant4/1 -> Divide2/2
  Divide2/1 -> Gain17/1
  in_D_PI/1(Out1) -> Goto10/1
  Gain17/1 -> in_D_PI/1(In1)

== system M10B39_es_V2/Genrators/Generator1 ==
  Vgxy : Inport
  Trip : Inport  Port=2
  Bistable2 : spsBistableLib/Bistable  Qpriority=Set  ic=0  Ts=0
      settings: LibrarySourceBlock=sps_lib/Control/Bistable
  Constant : Constant  Value=[0,0,0,0]
  Excitation System ST1A1 : Subsystem
  Governor : Subsystem
  Ground : Ground
  "Machine Equations " : Subsystem
  Mechanical DE : Subsystem
  Output : Subsystem
  PSS1 : Subsystem
  Scope{,1..3,5} (5 alike) : Scope
      Scope settings: ActiveDisplayYMinimum=-0.52997  ActiveDisplayYMaximum=12.90306  DataLoggingVariableName=ScopeData3
      Scope1 settings: ActiveDisplayYMinimum=7.63415  ActiveDisplayYMaximum=7.96859  DataLoggingVariableName=ScopeData2
      Scope2 settings: TimeSpan=10  ActiveDisplayYMinimum=-0.0003  ActiveDisplayYMaximum=0.0004  DataLoggingVariableName=ScopeData22
      Scope3 settings: TimeSpan=10  ActiveDisplayYMinimum=2.71193E-11  ActiveDisplayYMaximum=2.71256E-11  DataLoggingVariableName=ScopeData23
      Scope5 settings: TimeSpan=10  ActiveDisplayYMinimum=0.15  ActiveDisplayYMaximum=0.65  DataLoggingVariableName=ScopeData10
  Switch4 : Switch  Criteria=u2 ~= 0  Threshold=0.5  InputSameDT=off
  Terminator : Terminator
  pu->pu : Gain  Gain=SgenB./SgridB
  pu->pu1 : Gain  Gain=SgenB./SgridB
  m : Outport
  Igxy1 : Outport  Port=2
  GBxy : Outport  Port=3
  wires:
  pu->pu1/1 -> [GBxy]
  pu->pu/1 -> [Igxy1]
  "Machine Equations "/3(GBxy) -> Switch4/3
  Constant/1 -> Switch4/1
  Switch4/1 -> pu->pu1/1
  [Trip] -> Switch4/2
  [Trip] -> PSS1/2(Trip)
  [Trip] -> Governor/2(Trip)
  [Trip] -> Mechanical DE/3(Trip)
  [Trip] -> Excitation System ST1A1/2(Trip)
  [Trip] -> "Machine Equations "/4(Trip)
  Bistable2/2 -> Terminator/1
  Trip/1 -> Bistable2/1
  Ground/1 -> Bistable2/2
  Bistable2/1 -> [Trip]
  [Vg] -> Output/6(Vg)
  Output/1(m) -> m/1
  Output/3(GBxy) -> GBxy/1
  Output/2(Igxy1) -> Igxy1/1
  [Igxy1] -> Output/1(Igxy1in)
  [GBxy] -> Output/2(GBxyin)
  [delta] -> Output/3(deltain)
  [f] -> Output/5(fin)
  [Pe] -> Output/4(Pein)
  Mechanical DE/1(delta) -> "Machine Equations "/1(delta), [delta], Scope/1
  Governor/1(dPm) -> Scope3/1, Mechanical DE/2(dPm)
  PSS1/1(Upss) -> Scope2/1, Excitation System ST1A1/1(Upss)
  Mechanical DE/2(w) -> [f], PSS1/1(w), Governor/1(w)
  "Machine Equations "/2(Igxy1) -> pu->pu/1
  Vgxy/1 -> "Machine Equations "/2(Vgxy)
  "Machine Equations "/4(Vg) -> [Vg], Excitation System ST1A1/3(Vg)
  "Machine Equations "/1(Pe) -> [Pe], Mechanical DE/1(Pe), Scope1/1
  Excitation System ST1A1/1(Ef) -> "Machine Equations "/3(Ef), Scope5/1

== system M10B39_es_V2/Genrators/Generator10 ==
  Vgxy : Inport
  Trip : Inport  Port=2
  Bistable2 : spsBistableLib/Bistable  Qpriority=Set  ic=0  Ts=0
      settings: LibrarySourceBlock=sps_lib/Control/Bistable
  Constant : Constant  Value=[0,0,0,0]
  Excitation System ST1A1 : Subsystem
  Governor : Subsystem
  Ground : Ground
  "Machine Equations " : Subsystem
  Mechanical DE : Subsystem
  Output : Subsystem
  PSS1 : Subsystem
  Scope{,1..3,5} (5 alike) : Scope
      Scope settings: ActiveDisplayYMinimum=-0.52997  ActiveDisplayYMaximum=12.90306  DataLoggingVariableName=ScopeData3
      Scope1 settings: ActiveDisplayYMinimum=7.63415  ActiveDisplayYMaximum=7.96859  DataLoggingVariableName=ScopeData2
      Scope2 settings: TimeSpan=10  ActiveDisplayYMinimum=-0.0003  ActiveDisplayYMaximum=0.0004  DataLoggingVariableName=ScopeData22
      Scope3 settings: TimeSpan=10  ActiveDisplayYMinimum=2.71193E-11  ActiveDisplayYMaximum=2.71256E-11  DataLoggingVariableName=ScopeData23
      Scope5 settings: TimeSpan=10  ActiveDisplayYMinimum=0.15  ActiveDisplayYMaximum=0.65  DataLoggingVariableName=ScopeData10
  Switch4 : Switch  Criteria=u2 ~= 0  Threshold=0.5  InputSameDT=off
  Terminator : Terminator
  pu->pu : Gain  Gain=SgenB./SgridB
  pu->pu1 : Gain  Gain=SgenB./SgridB
  m : Outport
  Igxy1 : Outport  Port=2
  GBxy : Outport  Port=3
  wires:
  pu->pu1/1 -> [GBxy]
  pu->pu/1 -> [Igxy1]
  "Machine Equations "/3(GBxy) -> Switch4/3
  Constant/1 -> Switch4/1
  Switch4/1 -> pu->pu1/1
  [Trip] -> Switch4/2
  [Trip] -> PSS1/2(Trip)
  [Trip] -> Governor/2(Trip)
  [Trip] -> Mechanical DE/3(Trip)
  [Trip] -> Excitation System ST1A1/2(Trip)
  [Trip] -> "Machine Equations "/4(Trip)
  Bistable2/2 -> Terminator/1
  Trip/1 -> Bistable2/1
  Ground/1 -> Bistable2/2
  Bistable2/1 -> [Trip]
  [Vg] -> Output/6(Vg)
  Output/1(m) -> m/1
  Output/3(GBxy) -> GBxy/1
  Output/2(Igxy1) -> Igxy1/1
  [Igxy1] -> Output/1(Igxy1in)
  [GBxy] -> Output/2(GBxyin)
  [delta] -> Output/3(deltain)
  [f] -> Output/5(fin)
  [Pe] -> Output/4(Pein)
  Mechanical DE/1(delta) -> "Machine Equations "/1(delta), [delta], Scope/1
  Governor/1(dPm) -> Scope3/1, Mechanical DE/2(dPm)
  PSS1/1(Upss) -> Scope2/1, Excitation System ST1A1/1(Upss)
  Mechanical DE/2(w) -> [f], PSS1/1(w), Governor/1(w)
  "Machine Equations "/2(Igxy1) -> pu->pu/1
  Vgxy/1 -> "Machine Equations "/2(Vgxy)
  "Machine Equations "/4(Vg) -> [Vg], Excitation System ST1A1/3(Vg)
  "Machine Equations "/1(Pe) -> [Pe], Mechanical DE/1(Pe), Scope1/1
  Excitation System ST1A1/1(Ef) -> "Machine Equations "/3(Ef), Scope5/1

== system M10B39_es_V2/Genrators/Generator3 ==
  Vgxy : Inport
  Trip : Inport  Port=2
  Bistable2 : spsBistableLib/Bistable  Qpriority=Set  ic=0  Ts=0
      settings: LibrarySourceBlock=sps_lib/Control/Bistable
  Constant : Constant  Value=[0,0,0,0]
  Excitation System ST1A1 : Subsystem
  Governor : Subsystem
  Ground : Ground
  "Machine Equations " : Subsystem
  Mechanical DE : Subsystem
  Output : Subsystem
  PSS1 : Subsystem
  Scope{,1..3,5} (5 alike) : Scope
      Scope settings: ActiveDisplayYMinimum=-0.52997  ActiveDisplayYMaximum=12.90306  DataLoggingVariableName=ScopeData3
      Scope1 settings: ActiveDisplayYMinimum=7.63415  ActiveDisplayYMaximum=7.96859  DataLoggingVariableName=ScopeData2
      Scope2 settings: TimeSpan=10  ActiveDisplayYMinimum=-0.0003  ActiveDisplayYMaximum=0.0004  DataLoggingVariableName=ScopeData22
      Scope3 settings: TimeSpan=10  ActiveDisplayYMinimum=2.71193E-11  ActiveDisplayYMaximum=2.71256E-11  DataLoggingVariableName=ScopeData23
      Scope5 settings: TimeSpan=10  ActiveDisplayYMinimum=0.15  ActiveDisplayYMaximum=0.65  DataLoggingVariableName=ScopeData10
  Switch4 : Switch  Criteria=u2 ~= 0  Threshold=0.5  InputSameDT=off
  Terminator : Terminator
  pu->pu : Gain  Gain=SgenB./SgridB
  pu->pu1 : Gain  Gain=SgenB./SgridB
  m : Outport
  Igxy1 : Outport  Port=2
  GBxy : Outport  Port=3
  wires:
  pu->pu1/1 -> [GBxy]
  pu->pu/1 -> [Igxy1]
  "Machine Equations "/3(GBxy) -> Switch4/3
  Constant/1 -> Switch4/1
  Switch4/1 -> pu->pu1/1
  [Trip] -> Switch4/2
  [Trip] -> PSS1/2(Trip)
  [Trip] -> Governor/2(Trip)
  [Trip] -> Mechanical DE/3(Trip)
  [Trip] -> Excitation System ST1A1/2(Trip)
  [Trip] -> "Machine Equations "/4(Trip)
  Bistable2/2 -> Terminator/1
  Trip/1 -> Bistable2/1
  Ground/1 -> Bistable2/2
  Bistable2/1 -> [Trip]
  [Vg] -> Output/6(Vg)
  Output/1(m) -> m/1
  Output/3(GBxy) -> GBxy/1
  Output/2(Igxy1) -> Igxy1/1
  [Igxy1] -> Output/1(Igxy1in)
  [GBxy] -> Output/2(GBxyin)
  [delta] -> Output/3(deltain)
  [f] -> Output/5(fin)
  [Pe] -> Output/4(Pein)
  Mechanical DE/1(delta) -> "Machine Equations "/1(delta), [delta], Scope/1
  Governor/1(dPm) -> Scope3/1, Mechanical DE/2(dPm)
  PSS1/1(Upss) -> Scope2/1, Excitation System ST1A1/1(Upss)
  Mechanical DE/2(w) -> [f], PSS1/1(w), Governor/1(w)
  "Machine Equations "/2(Igxy1) -> pu->pu/1
  Vgxy/1 -> "Machine Equations "/2(Vgxy)
  "Machine Equations "/4(Vg) -> [Vg], Excitation System ST1A1/3(Vg)
  "Machine Equations "/1(Pe) -> [Pe], Mechanical DE/1(Pe), Scope1/1
  Excitation System ST1A1/1(Ef) -> "Machine Equations "/3(Ef), Scope5/1

== system M10B39_es_V2/Genrators/Generator4 ==
  Vgxy : Inport
  Trip : Inport  Port=2
  Bistable2 : spsBistableLib/Bistable  Qpriority=Set  ic=0  Ts=0
      settings: LibrarySourceBlock=sps_lib/Control/Bistable
  Constant : Constant  Value=[0,0,0,0]
  Excitation System ST1A1 : Subsystem
  Governor : Subsystem
  Ground : Ground
  "Machine Equations " : Subsystem
  Mechanical DE : Subsystem
  Output : Subsystem
  PSS1 : Subsystem
  Scope{,1..3,5} (5 alike) : Scope
      Scope settings: ActiveDisplayYMinimum=-0.52997  ActiveDisplayYMaximum=12.90306  DataLoggingVariableName=ScopeData3
      Scope1 settings: ActiveDisplayYMinimum=7.63415  ActiveDisplayYMaximum=7.96859  DataLoggingVariableName=ScopeData2
      Scope2 settings: TimeSpan=10  ActiveDisplayYMinimum=-0.0003  ActiveDisplayYMaximum=0.0004  DataLoggingVariableName=ScopeData22
      Scope3 settings: TimeSpan=10  ActiveDisplayYMinimum=2.71193E-11  ActiveDisplayYMaximum=2.71256E-11  DataLoggingVariableName=ScopeData23
      Scope5 settings: TimeSpan=10  ActiveDisplayYMinimum=0.15  ActiveDisplayYMaximum=0.65  DataLoggingVariableName=ScopeData10
  Switch4 : Switch  Criteria=u2 ~= 0  Threshold=0.5  InputSameDT=off
  Terminator : Terminator
  pu->pu : Gain  Gain=SgenB./SgridB
  pu->pu1 : Gain  Gain=SgenB./SgridB
  m : Outport
  Igxy1 : Outport  Port=2
  GBxy : Outport  Port=3
  wires:
  pu->pu1/1 -> [GBxy]
  pu->pu/1 -> [Igxy1]
  "Machine Equations "/3(GBxy) -> Switch4/3
  Constant/1 -> Switch4/1
  Switch4/1 -> pu->pu1/1
  [Trip] -> Switch4/2
  [Trip] -> PSS1/2(Trip)
  [Trip] -> Governor/2(Trip)
  [Trip] -> Mechanical DE/3(Trip)
  [Trip] -> Excitation System ST1A1/2(Trip)
  [Trip] -> "Machine Equations "/4(Trip)
  Bistable2/2 -> Terminator/1
  Trip/1 -> Bistable2/1
  Ground/1 -> Bistable2/2
  Bistable2/1 -> [Trip]
  [Vg] -> Output/6(Vg)
  Output/1(m) -> m/1
  Output/3(GBxy) -> GBxy/1
  Output/2(Igxy1) -> Igxy1/1
  [Igxy1] -> Output/1(Igxy1in)
  [GBxy] -> Output/2(GBxyin)
  [delta] -> Output/3(deltain)
  [f] -> Output/5(fin)
  [Pe] -> Output/4(Pein)
  Mechanical DE/1(delta) -> "Machine Equations "/1(delta), [delta], Scope/1
  Governor/1(dPm) -> Scope3/1, Mechanical DE/2(dPm)
  PSS1/1(Upss) -> Scope2/1, Excitation System ST1A1/1(Upss)
  Mechanical DE/2(w) -> [f], PSS1/1(w), Governor/1(w)
  "Machine Equations "/2(Igxy1) -> pu->pu/1
  Vgxy/1 -> "Machine Equations "/2(Vgxy)
  "Machine Equations "/4(Vg) -> [Vg], Excitation System ST1A1/3(Vg)
  "Machine Equations "/1(Pe) -> [Pe], Mechanical DE/1(Pe), Scope1/1
  Excitation System ST1A1/1(Ef) -> "Machine Equations "/3(Ef), Scope5/1

== system M10B39_es_V2/Genrators/Generator5 ==
  Vgxy : Inport
  Trip : Inport  Port=2
  Bistable2 : spsBistableLib/Bistable  Qpriority=Set  ic=0  Ts=0
      settings: LibrarySourceBlock=sps_lib/Control/Bistable
  Constant : Constant  Value=[0,0,0,0]
  Excitation System ST1A1 : Subsystem
  Governor : Subsystem
  Ground : Ground
  "Machine Equations " : Subsystem
  Mechanical DE : Subsystem
  Output : Subsystem
  PSS1 : Subsystem
  Scope{,1..3,5} (5 alike) : Scope
      Scope settings: ActiveDisplayYMinimum=-0.52997  ActiveDisplayYMaximum=12.90306  DataLoggingVariableName=ScopeData3
      Scope1 settings: ActiveDisplayYMinimum=7.63415  ActiveDisplayYMaximum=7.96859  DataLoggingVariableName=ScopeData2
      Scope2 settings: TimeSpan=10  ActiveDisplayYMinimum=-0.0003  ActiveDisplayYMaximum=0.0004  DataLoggingVariableName=ScopeData22
      Scope3 settings: TimeSpan=10  ActiveDisplayYMinimum=2.71193E-11  ActiveDisplayYMaximum=2.71256E-11  DataLoggingVariableName=ScopeData23
      Scope5 settings: TimeSpan=10  ActiveDisplayYMinimum=0.15  ActiveDisplayYMaximum=0.65  DataLoggingVariableName=ScopeData10
  Switch4 : Switch  Criteria=u2 ~= 0  Threshold=0.5  InputSameDT=off
  Terminator : Terminator
  pu->pu : Gain  Gain=SgenB./SgridB
  pu->pu1 : Gain  Gain=SgenB./SgridB
  m : Outport
  Igxy1 : Outport  Port=2
  GBxy : Outport  Port=3
  wires:
  pu->pu1/1 -> [GBxy]
  pu->pu/1 -> [Igxy1]
  "Machine Equations "/3(GBxy) -> Switch4/3
  Constant/1 -> Switch4/1
  Switch4/1 -> pu->pu1/1
  [Trip] -> Switch4/2
  [Trip] -> PSS1/2(Trip)
  [Trip] -> Governor/2(Trip)
  [Trip] -> Mechanical DE/3(Trip)
  [Trip] -> Excitation System ST1A1/2(Trip)
  [Trip] -> "Machine Equations "/4(Trip)
  Bistable2/2 -> Terminator/1
  Trip/1 -> Bistable2/1
  Ground/1 -> Bistable2/2
  Bistable2/1 -> [Trip]
  [Vg] -> Output/6(Vg)
  Output/1(m) -> m/1
  Output/3(GBxy) -> GBxy/1
  Output/2(Igxy1) -> Igxy1/1
  [Igxy1] -> Output/1(Igxy1in)
  [GBxy] -> Output/2(GBxyin)
  [delta] -> Output/3(deltain)
  [f] -> Output/5(fin)
  [Pe] -> Output/4(Pein)
  Mechanical DE/1(delta) -> "Machine Equations "/1(delta), [delta], Scope/1
  Governor/1(dPm) -> Scope3/1, Mechanical DE/2(dPm)
  PSS1/1(Upss) -> Scope2/1, Excitation System ST1A1/1(Upss)
  Mechanical DE/2(w) -> [f], PSS1/1(w), Governor/1(w)
  "Machine Equations "/2(Igxy1) -> pu->pu/1
  Vgxy/1 -> "Machine Equations "/2(Vgxy)
  "Machine Equations "/4(Vg) -> [Vg], Excitation System ST1A1/3(Vg)
  "Machine Equations "/1(Pe) -> [Pe], Mechanical DE/1(Pe), Scope1/1
  Excitation System ST1A1/1(Ef) -> "Machine Equations "/3(Ef), Scope5/1

== system M10B39_es_V2/Genrators/Generator7 ==
  Vgxy : Inport
  Trip : Inport  Port=2
  Bistable2 : spsBistableLib/Bistable  Qpriority=Set  ic=0  Ts=0
      settings: LibrarySourceBlock=sps_lib/Control/Bistable
  Constant : Constant  Value=[0,0,0,0]
  Excitation System ST1A1 : Subsystem
  Governor : Subsystem
  Ground : Ground
  "Machine Equations " : Subsystem
  Mechanical DE : Subsystem
  Output : Subsystem
  PSS1 : Subsystem
  Scope{,1..3,5} (5 alike) : Scope
      Scope settings: ActiveDisplayYMinimum=-0.52997  ActiveDisplayYMaximum=12.90306  DataLoggingVariableName=ScopeData3
      Scope1 settings: ActiveDisplayYMinimum=7.63415  ActiveDisplayYMaximum=7.96859  DataLoggingVariableName=ScopeData2
      Scope2 settings: TimeSpan=10  ActiveDisplayYMinimum=-0.0003  ActiveDisplayYMaximum=0.0004  DataLoggingVariableName=ScopeData22
      Scope3 settings: TimeSpan=10  ActiveDisplayYMinimum=2.71193E-11  ActiveDisplayYMaximum=2.71256E-11  DataLoggingVariableName=ScopeData23
      Scope5 settings: TimeSpan=10  ActiveDisplayYMinimum=0.15  ActiveDisplayYMaximum=0.65  DataLoggingVariableName=ScopeData10
  Switch4 : Switch  Criteria=u2 ~= 0  Threshold=0.5  InputSameDT=off
  Terminator : Terminator
  pu->pu : Gain  Gain=SgenB./SgridB
  pu->pu1 : Gain  Gain=SgenB./SgridB
  m : Outport
  Igxy1 : Outport  Port=2
  GBxy : Outport  Port=3
  wires:
  pu->pu1/1 -> [GBxy]
  pu->pu/1 -> [Igxy1]
  "Machine Equations "/3(GBxy) -> Switch4/3
  Constant/1 -> Switch4/1
  Switch4/1 -> pu->pu1/1
  [Trip] -> Switch4/2
  [Trip] -> PSS1/2(Trip)
  [Trip] -> Governor/2(Trip)
  [Trip] -> Mechanical DE/3(Trip)
  [Trip] -> Excitation System ST1A1/2(Trip)
  [Trip] -> "Machine Equations "/4(Trip)
  Bistable2/2 -> Terminator/1
  Trip/1 -> Bistable2/1
  Ground/1 -> Bistable2/2
  Bistable2/1 -> [Trip]
  [Vg] -> Output/6(Vg)
  Output/1(m) -> m/1
  Output/3(GBxy) -> GBxy/1
  Output/2(Igxy1) -> Igxy1/1
  [Igxy1] -> Output/1(Igxy1in)
  [GBxy] -> Output/2(GBxyin)
  [delta] -> Output/3(deltain)
  [f] -> Output/5(fin)
  [Pe] -> Output/4(Pein)
  Mechanical DE/1(delta) -> "Machine Equations "/1(delta), [delta], Scope/1
  Governor/1(dPm) -> Scope3/1, Mechanical DE/2(dPm)
  PSS1/1(Upss) -> Scope2/1, Excitation System ST1A1/1(Upss)
  Mechanical DE/2(w) -> [f], PSS1/1(w), Governor/1(w)
  "Machine Equations "/2(Igxy1) -> pu->pu/1
  Vgxy/1 -> "Machine Equations "/2(Vgxy)
  "Machine Equations "/4(Vg) -> [Vg], Excitation System ST1A1/3(Vg)
  "Machine Equations "/1(Pe) -> [Pe], Mechanical DE/1(Pe), Scope1/1
  Excitation System ST1A1/1(Ef) -> "Machine Equations "/3(Ef), Scope5/1
